simulink model "Erreur_RegimePermanent"  (R2025b)
settings: Solver=VariableStepAuto  StartTime=0.0  StopTime=600  RelTol=1e-3
values from neighbouring files (symbols this model uses):
  Kd = 0.01    [Dev_04_M.m]
  Ki = 0.1    [Dev_04_M.m]
  Kp = 5    [Dev_04_M.m]
settings Model: Creator=Louis  LastModifiedBy=Louis

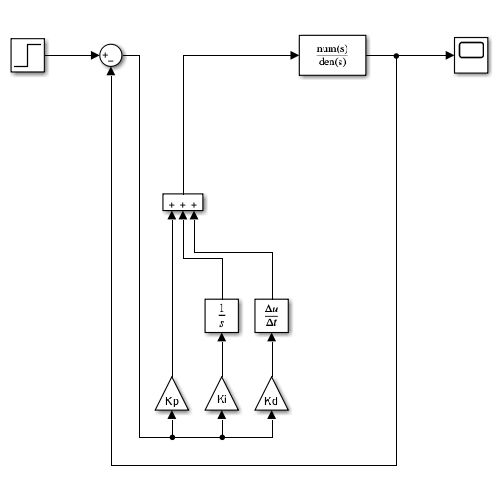
[thumbnail: Simulink's stored preview of the top-level diagram]
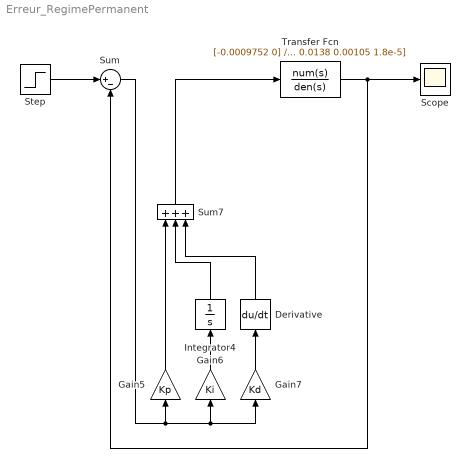
== system Erreur_RegimePermanent ==
  Derivative : Derivative
  Gain5 : Gain  Gain=Kp
  Gain6 : Gain  Gain=Ki
  Gain7 : Gain  Gain=Kd
  Integrator4 : Integrator
  Scope : Scope
      settings: ActiveDisplayYMinimum=-278.99047648394685  ActiveDisplayYMaximum=140.3932392891856
  Step : Step  Time=0  After=2  SampleTime=0
  Sum : Sum  Inputs=|+-
  Sum7 : Sum  Inputs=+++
  Transfer Fcn : TransferFcn  Numerator=[-0.0009752 0]  Denominator=[1 0.335 0.0138 0.00105 1.8e-5]
  wires:
  Gain5/1 -> Sum7/1
  Derivative/1 -> Sum7/3
  Gain6/1 -> Integrator4/1
  Integrator4/1 -> Sum7/2
  Gain7/1 -> Derivative/1
  Step/1 -> Sum/1
  Sum/1 -> Gain7/1, Gain6/1, Gain5/1
  Transfer Fcn/1 -> Sum/2, Scope/1
  Sum7/1 -> Transfer Fcn/1
